simulink model "wopwop"  (R2013b)
settings: Solver=ode45  StartTime=0.0  StopTime=10.0  RelTol=1e-3
undefined symbols (not defined in the file): Hb, K, Kd, Ki, Kp, T
settings Model: Creator=nickoe  LastModifiedBy=jeppe
settings DebuggingCC: StateNameClashWarn=warning

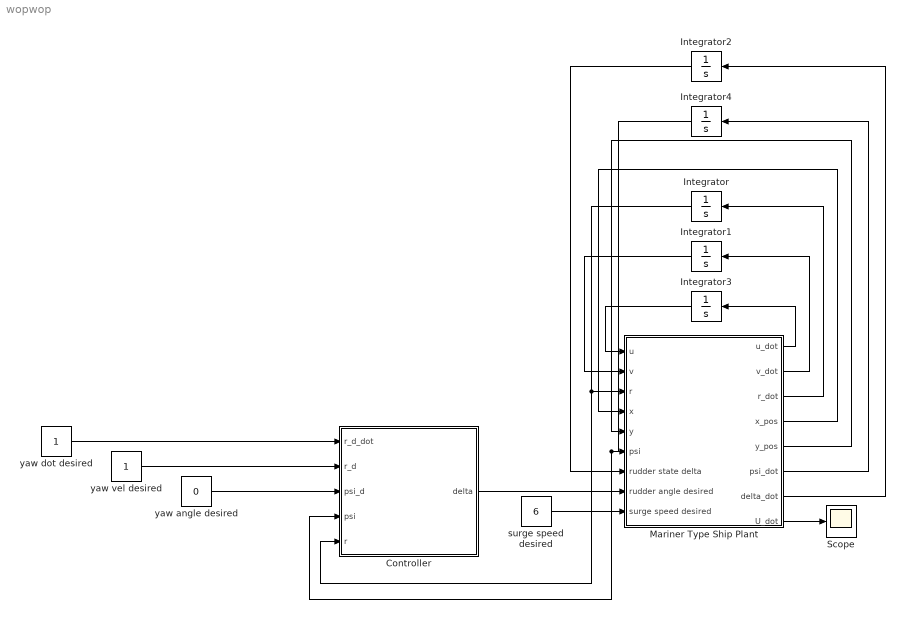
== system wopwop ==
  Controller : Subsystem  InitFcn=load('modelParameters.mat')
  Integrator{,1..4} (5 alike) : Integrator
  Mariner Type Ship Plant : Subsystem
  Scope : Scope
  surge speed desired : Constant  Value=6
  yaw angle desired : Constant  Value=0
  yaw dot desired : Constant
  yaw vel desired : Constant
  wires:
  surge speed desired/1 -> Mariner Type Ship Plant/9(surge speed desired)
  Controller/1(delta) -> Mariner Type Ship Plant/8(rudder angle desired)
  Mariner Type Ship Plant/3(r_dot) -> Integrator/1
  Mariner Type Ship Plant/6(psi_dot) -> Integrator4/1
  Mariner Type Ship Plant/1(u_dot) -> Integrator3/1
  Mariner Type Ship Plant/2(v_dot) -> Integrator1/1
  Mariner Type Ship Plant/7(delta_dot) -> Integrator2/1
  Integrator3/1 -> Mariner Type Ship Plant/1(u)
  Integrator4/1 -> Controller/4(psi), Mariner Type Ship Plant/6(psi)
  Integrator2/1 -> Mariner Type Ship Plant/7(rudder state delta)
  Mariner Type Ship Plant/4(x_pos) -> Mariner Type Ship Plant/4(x)
  Integrator/1 -> Controller/5(r), Mariner Type Ship Plant/3(r)
  Integrator1/1 -> Mariner Type Ship Plant/2(v)
  yaw angle desired/1 -> Controller/3(psi_d)
  yaw vel desired/1 -> Controller/2(r_d)
  yaw dot desired/1 -> Controller/1(r_d_dot)
  Mariner Type Ship Plant/5(y_pos) -> Mariner Type Ship Plant/5(y)
  Mariner Type Ship Plant/8(U_dot) -> Scope/1

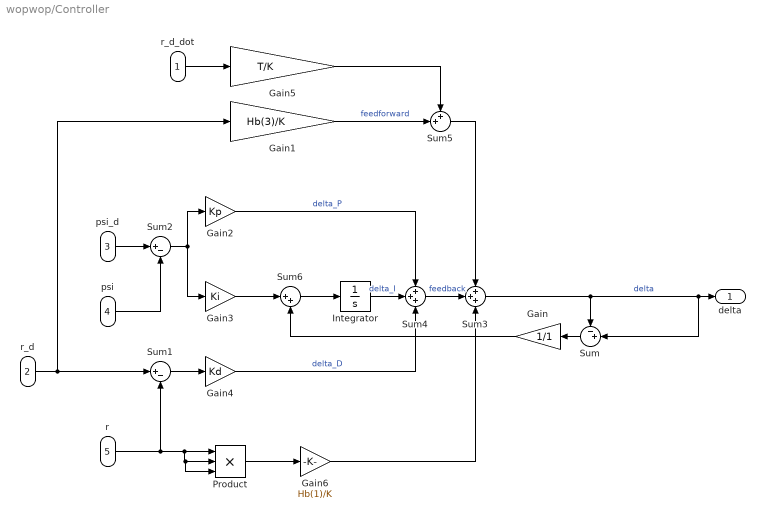
== system wopwop/Controller ==
  r_d_dot : Inport
  r_d : Inport  Port=2
  psi_d : Inport  Port=3
  psi : Inport  Port=4
  r : Inport  Port=5
  Gain : Gain  Gain=1/1
  Gain1 : Gain  Gain=Hb(3)/K
  Gain2 : Gain  Gain=Kp
  Gain3 : Gain  Gain=Ki
  Gain4 : Gain  Gain=Kd
  Gain5 : Gain  Gain=T/K
  Gain6 : Gain  Gain=Hb(1)/K
  Integrator : Integrator
  Product : Product  Inputs=3  RndMeth=Zero
  Sum : Sum  Inputs=-+|
  Sum1 : Sum  Inputs=|+-
  Sum2 : Sum  Inputs=|+-
  Sum3 : Sum  Inputs=+++
  Sum4 : Sum  Inputs=+++
  Sum5 : Sum  Inputs=++|
  Sum6 : Sum  Inputs=|++
  delta : Outport
  wires:
  Gain4/1 -> Sum4/3  "delta_D"
  Gain2/1 -> Sum4/1  "delta_P"
  Integrator/1 -> Sum4/2  "delta_I"
  r_d/1 -> Gain1/1, Sum1/1
  Sum1/1 -> Gain4/1
  r/1 -> Sum1/2, Product/3, Product/2, Product/1
  Sum2/1 -> Gain3/1, Gain2/1
  psi/1 -> Sum2/2
  psi_d/1 -> Sum2/1
  Sum3/1 -> Sum/1, Sum/2, delta/1  "delta"
  Sum4/1 -> Sum3/2  "feedback"
  Gain1/1 -> Sum5/2  "feedforward"
  Sum5/1 -> Sum3/1
  r_d_dot/1 -> Gain5/1
  Gain5/1 -> Sum5/1
  Sum/1 -> Gain/1
  Sum6/1 -> Integrator/1
  Gain3/1 -> Sum6/1
  Gain/1 -> Sum6/2
  Product/1 -> Gain6/1
  Gain6/1 -> Sum3/3

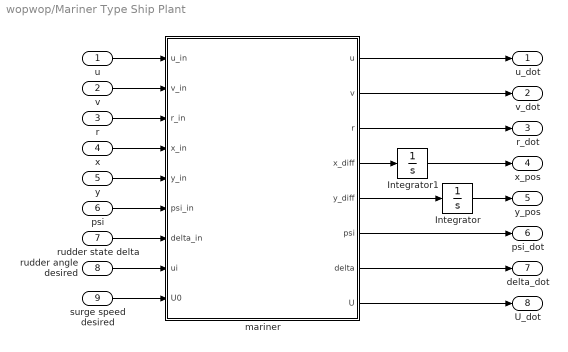
== system wopwop/Mariner Type Ship Plant ==
  u : Inport
  v : Inport  Port=2
  r : Inport  Port=3
  x : Inport  Port=4
  y : Inport  Port=5
  psi : Inport  Port=6
  rudder state delta : Inport  Port=7
  rudder angle desired : Inport  Port=8
  surge speed desired : Inport  Port=9
  Integrator : Integrator
  Integrator1 : Integrator
  mariner : MATLAB Function  TreatAsAtomicUnit=on
  u_dot : Outport
  v_dot : Outport  Port=2
  r_dot : Outport  Port=3
  x_pos : Outport  Port=4
  y_pos : Outport  Port=5
  psi_dot : Outport  Port=6
  delta_dot : Outport  Port=7
  U_dot : Outport  Port=8
  wires:
  Integrator/1 -> y_pos/1
  mariner/5(y_diff) -> Integrator/1
  Integrator1/1 -> x_pos/1
  mariner/8(U) -> U_dot/1
  mariner/6(psi) -> psi_dot/1
  mariner/4(x_diff) -> Integrator1/1
  u/1 -> mariner/1(u_in)
  mariner/7(delta) -> delta_dot/1
  mariner/1(u) -> u_dot/1
  mariner/2(v) -> v_dot/1
  mariner/3(r) -> r_dot/1
  v/1 -> mariner/2(v_in)
  r/1 -> mariner/3(r_in)
  x/1 -> mariner/4(x_in)
  y/1 -> mariner/5(y_in)
  psi/1 -> mariner/6(psi_in)
  rudder state delta/1 -> mariner/7(delta_in)
  rudder angle desired/1 -> mariner/8(ui)
  surge speed desired/1 -> mariner/9(U0)

== matlab function wopwop/Mariner Type Ship Plant/mariner ==
  data: u_in input; v_in input; r_in input; x_in input; y_in input; psi_in input; delta_in input; u output; v output; r output; x_diff output; y_diff output; psi output; delta output; ui input; U0 input; U output
function [u,v,r,x_diff,y_diff,psi,delta,U] = fcn( u_in,v_in,r_in,x_in,y_in,psi_in,delta_in, ui,U0)
%#codegen
xdot = zeros(1,7);
[xdot,U] = mariner([u_in,v_in,r_in,x_in,y_in,psi_in,delta_in],ui,U0);
u = xdot(1);
v = xdot(2);
r = xdot(3);
x_diff = xdot(4);
y_diff = xdot(5);
psi = xdot(6);
delta = xdot(7);
end
